simulink model "algeb2"  (Simulink 4.00)
settings: Solver=ode45  StartTime=0.0  StopTime=10.0  RelTol=1e-3
libraries: simulink3 x1
settings Model: LastModifiedBy=Administrator  BlockReductionOpt=off

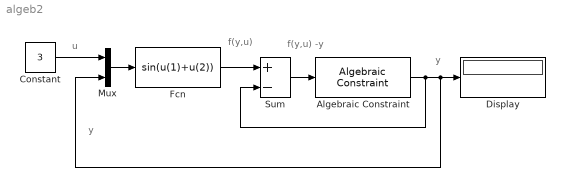
== system algeb2 ==
  note: u
  note: y
  note: f(y,u)
  note: y
  note: f(y,u) -y
  Algebraic Constraint : simulink3/Math/Algebraic Constraint  z0=0
  Constant : Constant  Value=3
  Display : Display
      settings: Format=short
  Fcn : Fcn  Expr=sin(u(1)+u(2))
  Mux : Mux  Inputs=2
  Sum : Sum  Inputs=+-  SaturateOnIntegerOverflow=on
  wires:
  Constant/1 -> Mux/1
  Mux/1 -> Fcn/1
  Fcn/1 -> Sum/1
  Sum/1 -> Algebraic Constraint/1
  Algebraic Constraint/1 -> Sum/2, Mux/2, Display/1
